simulink model "guidance"  (R2020b)
settings: Solver=FixedStepAuto  StartTime=0.0  StopTime=inf  FixedStep=0.01  RelTol=1e-3
settings Model: DataDictionary=kspdemo.sldd  EnablePacing=on  PacingRate=2  Creator=brianhannan  LastModifiedBy=bhannan

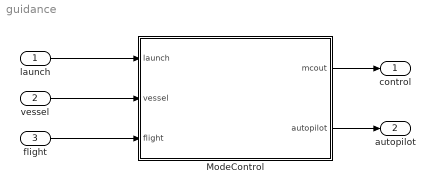
== system guidance ==
  launch : Inport  OutDataTypeStr=boolean  PortDimensions=1
  vessel : Inport  Port=2  OutDataTypeStr=Bus: vesselRx
  flight : Inport  Port=3  OutDataTypeStr=Bus: flight
  ModeControl : Subsystem  mask(FlightMode){}
      mask help: Flight mode state machine. Performs high-level mission logic (launch, staging, etc.).
      mask Display:
      | disp('Flight Mode')
      | 
      | port_label('input',1,'launch')
      | port_label('input',2,'vessel')
      | port_label('input',3,'flight')
      | 
      | port_label('output',1,'control')
      | port_label('output',2,'autopilot')
  control : Outport  OutDataTypeStr=Bus: mcout
  autopilot : Outport  Port=2  OutDataTypeStr=Bus: autopilot
  wires:
  launch/1 -> ModeControl/1(launch)
  ModeControl/1(mcout) -> control/1
  ModeControl/2(autopilot) -> autopilot/1
  vessel/1 -> ModeControl/2(vessel)
  flight/1 -> ModeControl/3(flight)

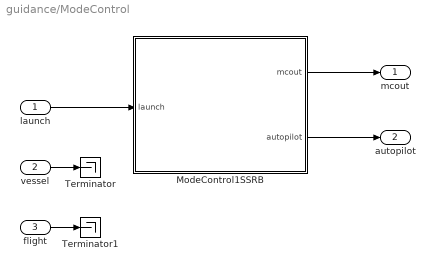
== system guidance/ModeControl ==
  launch : Inport
  vessel : Inport  Port=2
  flight : Inport  Port=3
  ModeControl1SSRB : Stateflow chart  TreatAsAtomicUnit=on  mask(ModeControl){}
      mask help: Mode control
  Terminator : Terminator
  Terminator1 : Terminator
  mcout : Outport
  autopilot : Outport  Port=2
  wires:
  flight/1 -> Terminator1/1
  vessel/1 -> Terminator/1
  ModeControl1SSRB/1(mcout) -> mcout/1
  launch/1 -> ModeControl1SSRB/1(launch)
  ModeControl1SSRB/2(autopilot) -> autopilot/1

== stateflow chart guidance/ModeControl/ModeControl1SSRB ==
  state Prelaunch
    en:
    mcout.mode = int8(-100);
    autopilot.targetPitch = 90;
    autopilot.targetHeading = 90;
    autopilot.engage = true;
  state Launch
    en:
    mcout.mode = int8(0);
    state PreFlightChecks
      en:
      % to do: add prelaunch check logic
      launchChecksOK = true;
    (default) -> PreFlightChecks
  state Stage1
    en:
    mcout.mode = int8(100);
    du:
    if ~launchCmdSent
    mcout.activateNextStage = true;
    launchCmdSent = true;
    else
    mcout.activateNextStage = false;
    end
  state SRBSeparation
    en:
    mcout.mode = int8(200);
    du:
    if ~stage1sepCmdSent
    mcout.activateNextStage = true;
    stage1sepCmdSent = true;
    else
    mcout.activateNextStage = false;
    end
  (default) -> Prelaunch
  Prelaunch -> Launch : [launch == true]
  Launch -> (junction 31) [order 1] : [launchChecksOK == true]
  (junction 31) -> Stage1 : [after(0.5,sec)]
  Stage1 -> (junction 27)
  (junction 27) -> SRBSeparation [order 1] : [t>inf]
  (junction 27) -> (junction 29) [order 2]
  Launch -> Prelaunch [order 2] : [launchChecksOK == false]
  data: launch input boolean size=1; mcout output Bus: mcout size=1; launchChecksOK local boolean =true; autopilot output Bus: autopilot; stage1sepCmdSent local boolean =false; launchCmdSent local boolean =false
